simulink model "usbserial"  (R2022b)
settings: Solver=FixedStepDiscrete  StartTime=0.0  StopTime=inf  FixedStep=0.1  RelTol=1e-3
libraries: teensy_lib x2
settings Model: Creator=LabUser  LastModifiedBy=stefa
settings OptimizationCC: ReuseModelBlockBuffer=on  EnhancedBackFolding=on  PassReuseOutputArgsAs=Individual arguments  ZeroExternalMemoryAtStartup=off  ZeroInternalMemoryAtStartup=off  OptimizeBlockOrder=speed  DifferentSizesBufferReuse=on  OptimizationCustomize=off  EfficientTunableParamExpr=on
settings DebuggingCC: ParameterTunabilityLossMsg=error
settings HardwareCC: ProdBitPerPointer=32  ProdBitPerSizeT=32  ProdBitPerPtrDiffT=32  ProdLargestAtomicInteger=Long  ProdLargestAtomicFloat=Double  ProdWordSize=32  ProdHWDeviceType=ARM Compatible->ARM Cortex-M
settings SFSimCC: MATLABDynamicMemAlloc=off
settings RTWCC: Description=Teensy ERT Target  SystemTargetFile=teensy_ert.tlc  TemplateMakefile=teensy_ert.tmf  TargetLang=C++
settings CodeAppCC: ForceParamTrailComments=on  IgnoreCustomStorageClasses=off  OperatorAnnotations=on  SimulinkDataObjDesc=on  SFDataObjDesc=on  InsertBlockDesc=on
settings STFCustomTargetCC: TargetLibSuffix=.a  TargetLangStandard=C++11 (ISO)  MultiwordLength=256  GenerateSampleERTMain=on  CombineOutputUpdateFcns=on  ERTCustomFileBanners=on  SupportContinuousTime=off  SupportNonInlinedSFcns=off  RemoveResetFunc=on  MATLABClassNameForMDSCustomization=Simulink.SoftwareTarget.ERTCustomization  CPPClassGenCompliant=on  SystemTargetFile=teensy_ert.tlc
settings ERTTargetCC: TargetLangStandard=C++11 (ISO)  GenerateSampleERTMain=on  ParMdlRefBuildCompliant=off  CompOptLevelCompliant=off  ConcurrentExecutionCompliant=off  ModelStepFunctionPrototypeControlCompliant=off  UseToolchainInfoCompliant=off  ExtModeTransport=1  ExtModeMexFile=ext_serial_win32_comm  ExtModeMexArgs=0 5 4000000  ERTCustomFileTemplate=teensy_ert_file_process.tlc

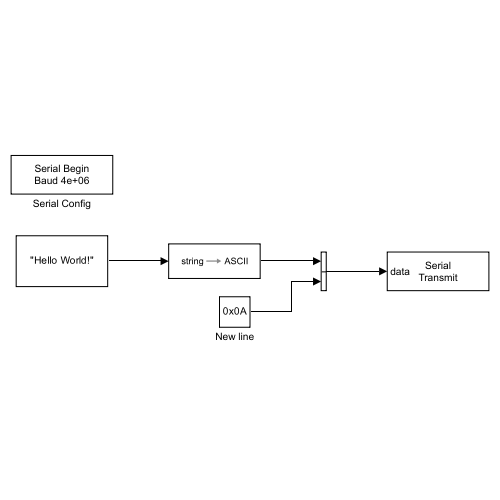
[thumbnail: Simulink's stored preview of the top-level diagram]
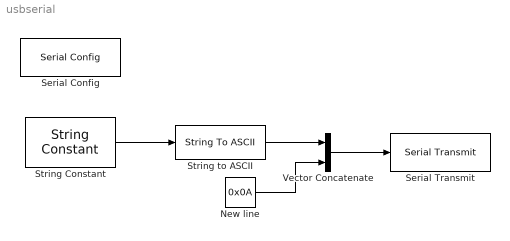
== system usbserial ==
  New line : Constant  Value=0x0A  OutDataTypeStr=uint8
  Serial Config : teensy_lib/Serial Config  SParameter1=Serial  SParameter2=4000000  SParameter3=10
      settings: SourceProductName=Custom C/C++ Target - Teensy
  Serial Transmit : teensy_lib/Serial Transmit  SParameter1=Serial  SampleTime=-1
      settings: SourceProductName=Custom C/C++ Target - Teensy
  String Constant : StringConstant  String="\"Hello World!\""
  String to ASCII : StringToASCII
  Vector Concatenate : Concatenate
  wires:
  String Constant/1 -> String to ASCII/1
  String to ASCII/1 -> Vector Concatenate/1
  Vector Concatenate/1 -> Serial Transmit/1
  New line/1 -> Vector Concatenate/2
